simulink model "Controllers"  (R2024a)
settings: Solver=VariableStepAuto  StartTime=0.0  StopTime=10.0  RelTol=1e-3
undefined symbols (not defined in the file): Earth, gains, initcond, params, WGS84
libraries: ArdupilotFunctions x7, aerolibtransform2 x1, sharedtransform x1
settings Model: Creator=igmso  LastModifiedBy=igmso

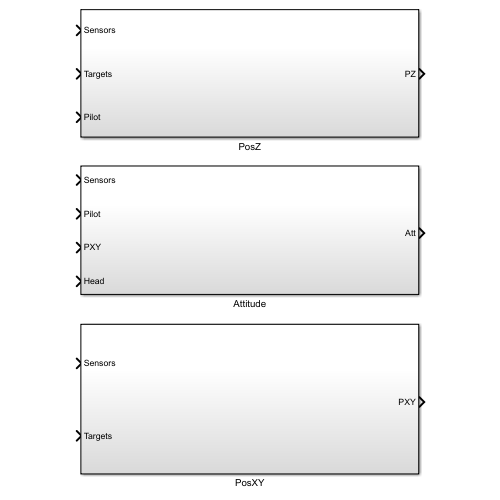
[thumbnail: Simulink's stored preview of the top-level diagram]
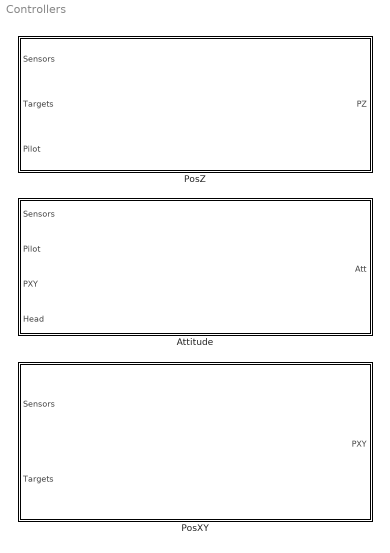
== system Controllers ==
  Attitude : Subsystem
  PosXY : Subsystem
  PosZ : Subsystem

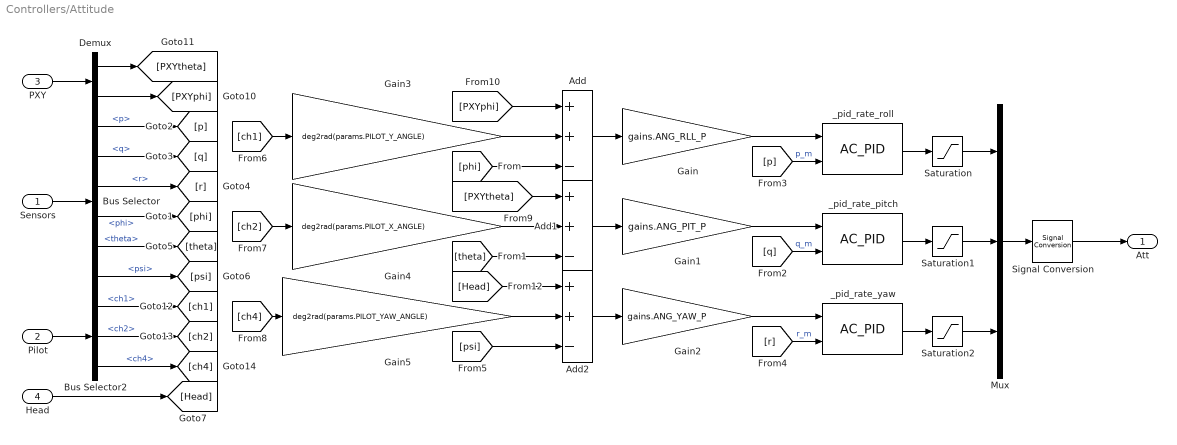
== system Controllers/Attitude ==
  Sensors : Inport  OutDataTypeStr=Bus: sensorsBus  PortDimensions=1
  Pilot : Inport  Port=2  OutDataTypeStr=Bus: pilotBus  PortDimensions=1
  PXY : Inport  Port=3  OutDataTypeStr=double  PortDimensions=2
  Head : Inport  Port=4  OutDataTypeStr=double  PortDimensions=1
  Add : Sum  Inputs=++-
  Add1 : Sum  Inputs=++-
  Add2 : Sum  Inputs=++-
  Bus Selector : BusSelector  OutputSignals=p,q,r,phi,theta,psi
  Bus Selector2 : BusSelector  OutputSignals=ch1,ch2,ch4
  Demux : Demux  Outputs=2
  Gain : Gain  Gain=gains.ANG_RLL_P
  Gain1 : Gain  Gain=gains.ANG_PIT_P
  Gain2 : Gain  Gain=gains.ANG_YAW_P
  Gain3 : Gain  Gain=deg2rad(params.PILOT_Y_ANGLE)
  Gain4 : Gain  Gain=deg2rad(params.PILOT_X_ANGLE)
  Gain5 : Gain  Gain=deg2rad(params.PILOT_YAW_ANGLE)
  Mux : Mux  Inputs=3
  Saturation : Saturate  UpperLimit=1  LowerLimit=-1
  Saturation1 : Saturate  UpperLimit=1  LowerLimit=-1
  Saturation2 : Saturate  UpperLimit=1  LowerLimit=-1
  Signal Conversion : SignalConversion  OverrideOpt=off
  _pid_rate_pitch : ArdupilotFunctions/AC_PID  P=gains.RAT_PIT_P  I=gains.RAT_PIT_I  D=gains.RAT_PIT_D  FF=gains.RAT_PIT_FF  D_FF=gains.RAT_PIT_D_FF  FLTD=gains.RAT_PIT_FLTD  FLTE=gains.RAT_PIT_FLTE  FLTT=gains.RAT_PIT_FLTT  IMAX=gains.RAT_PIT_IMAX  ControlFreq=rates.AttControl
  _pid_rate_roll : ArdupilotFunctions/AC_PID  P=gains.RAT_RLL_P  I=gains.RAT_RLL_I  D=gains.RAT_RLL_D  FF=gains.RAT_RLL_FF  D_FF=gains.RAT_RLL_D_FF  FLTD=gains.RAT_RLL_FLTD  FLTE=gains.RAT_RLL_FLTE  FLTT=gains.RAT_RLL_FLTT  IMAX=gains.RAT_RLL_IMAX  ControlFreq=rates.AttControl
  _pid_rate_yaw : ArdupilotFunctions/AC_PID  P=gains.RAT_YAW_P  I=gains.RAT_YAW_I  D=gains.RAT_YAW_D  FF=gains.RAT_YAW_FF  D_FF=gains.RAT_YAW_D_FF  FLTD=gains.RAT_YAW_FLTD  FLTE=gains.RAT_YAW_FLTE  FLTT=gains.RAT_YAW_FLTT  IMAX=gains.RAT_YAW_IMAX  ControlFreq=rates.AttControl
  Att : Outport  PortDimensions=3
  wires:
  Demux/1 -> [PXYtheta]
  _pid_rate_pitch/1 -> Saturation1/1
  Bus Selector2/3 -> [ch4]  "<ch4>"
  [ch2] -> Gain4/1
  Gain5/1 -> Add2/2
  Head/1 -> [Head]
  Bus Selector/2 -> [q]  "<q>"
  _pid_rate_roll/1 -> Saturation/1
  PXY/1 -> Demux/1
  [phi] -> Add/3
  Bus Selector/3 -> [r]  "<r>"
  [PXYtheta] -> Add1/1
  Bus Selector/5 -> [theta]  "<theta>"
  [Head] -> Add2/1
  Bus Selector/4 -> [phi]  "<phi>"
  Saturation2/1 -> Mux/3
  Gain4/1 -> Add1/2
  Mux/1 -> Signal Conversion/1
  [ch1] -> Gain3/1
  Gain2/1 -> _pid_rate_yaw/1
  Add2/1 -> Gain2/1
  [theta] -> Add1/3
  Signal Conversion/1 -> Att/1
  [q] -> _pid_rate_pitch/2  "q_m"
  Gain1/1 -> _pid_rate_pitch/1
  [p] -> _pid_rate_roll/2  "p_m"
  [r] -> _pid_rate_yaw/2  "r_m"
  [PXYphi] -> Add/1
  Add/1 -> Gain/1
  Sensors/1 -> Bus Selector/1
  [ch4] -> Gain5/1
  Gain3/1 -> Add/2
  Pilot/1 -> Bus Selector2/1
  Bus Selector/6 -> [psi]  "<psi>"
  Bus Selector/1 -> [p]  "<p>"
  Add1/1 -> Gain1/1
  Demux/2 -> [PXYphi]
  Saturation1/1 -> Mux/2
  _pid_rate_yaw/1 -> Saturation2/1
  Gain/1 -> _pid_rate_roll/1
  [psi] -> Add2/3
  Bus Selector2/2 -> [ch2]  "<ch2>"
  Bus Selector2/1 -> [ch1]  "<ch1>"
  Saturation/1 -> Mux/1

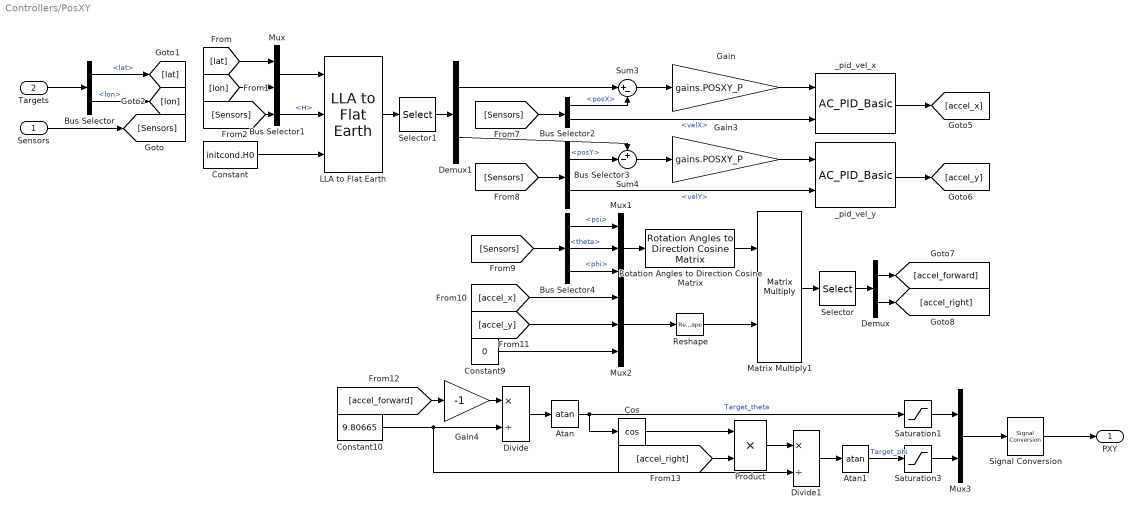
== system Controllers/PosXY ==
  Sensors : Inport  OutDataTypeStr=Bus: sensorsBus  PortDimensions=1
  Targets : Inport  Port=2  OutDataTypeStr=Bus: targetsBus  PortDimensions=1
  Atan : Trigonometry  Operator=atan
  Atan1 : Trigonometry  Operator=atan
  Bus Selector : BusSelector  OutputSignals=lat,lon
  Bus Selector1 : BusSelector  OutputSignals=H
  Bus Selector2 : BusSelector  OutputSignals=posX,velX
  Bus Selector3 : BusSelector  OutputSignals=posY,velY
  Bus Selector4 : BusSelector  OutputSignals=psi,theta,phi
  Constant : Constant  Value=initcond.H0  SampleTime=-1
  Constant10 : Constant  Value=9.80665  SampleTime=-1
  Constant9 : Constant  Value=0  SampleTime=-1
  Cos : Trigonometry  Operator=cos
  Demux : Demux  Outputs=2
  Demux1 : Demux  Outputs=2
  Divide : Product  Inputs=*/
  Divide1 : Product  Inputs=*/
  Gain : Gain  Gain=gains.POSXY_P
  Gain3 : Gain  Gain=gains.POSXY_P
  Gain4 : Gain  Gain=-1
  LLA to Flat Earth : aerolibtransform2/LLA to Flat Earth  units=Metric (MKS)  ptype=Earth (WGS84)  F=1/298.257223563  R=6378137  refPosPort=off  LL0=[0 10]  psi=0
  Matrix Multiply1 : Product  Multiplication=Matrix(*)
  Mux : Mux  Inputs=2
  Mux1 : Mux  Inputs=3
  Mux2 : Mux  Inputs=3
  Mux3 : Mux  Inputs=2
  Product : Product
  Reshape : Reshape  OutputDimensionality=Column vector (2-D)
  Rotation Angles to Direction Cosine Matrix : sharedtransform/Rotation Angles to Direction Cosine Matrix  rotationOrder=ZYX  aMode=aMode
  Saturation1 : Saturate  UpperLimit=deg2rad(gains.ANGLE_MAX)  LowerLimit=-deg2rad(gains.ANGLE_MAX)
  Saturation3 : Saturate
  Selector : Selector  InputPortWidth=3  IndexOptions=Index vector (dialog)  Indices=[1 2]  OutputSizes=1
  Selector1 : Selector  InputPortWidth=3  IndexOptions=Index vector (dialog)  Indices=[1 2]  OutputSizes=1
  Signal Conversion : SignalConversion  OverrideOpt=off
  Sum3 : Sum  Inputs=|+-
  Sum4 : Sum  Inputs=+-|
  _pid_vel_x : ArdupilotFunctions/AC_PID_Basic  P=gains.VELXY_P  I=gains.VELXY_I  D=gains.VELXY_D  FF=gains.VELXY_FF  FLTD=gains.VELXY_FLTD  FLTE=gains.VELXY_FLTE  IMAX=gains.VELXY_IMAX  ControlFreq=rates.PosControl
  _pid_vel_y : ArdupilotFunctions/AC_PID_Basic  P=gains.VELXY_P  I=gains.VELXY_I  D=gains.VELXY_D  FF=gains.VELXY_FF  FLTD=gains.VELXY_FLTD  FLTE=gains.VELXY_FLTE  IMAX=gains.VELXY_IMAX  ControlFreq=rates.PosControl
  PXY : Outport  PortDimensions=2
  wires:
  Reshape/1 -> Matrix Multiply1/2
  Saturation3/1 -> Mux3/2
  Divide/1 -> Atan/1
  Bus Selector/2 -> [lon]  "<lon>"
  Demux1/1 -> Sum3/1
  Sum3/1 -> Gain/1
  Bus Selector4/3 -> Mux1/3  "<phi>"
  Targets/1 -> Bus Selector/1
  Selector1/1 -> Demux1/1
  [Sensors] -> Bus Selector1/1
  _pid_vel_y/1 -> [accel_y]
  Product/1 -> Divide1/1
  Selector/1 -> Demux/1
  [Sensors] -> Bus Selector4/1
  Demux1/2 -> Sum4/1
  Gain/1 -> _pid_vel_x/1
  Mux1/1 -> Rotation Angles to Direction Cosine Matrix/1
  Sum4/1 -> Gain3/1
  Bus Selector3/2 -> _pid_vel_y/2  "<velY>"
  Bus Selector1/1 -> LLA to Flat Earth/2  "<H>"
  Divide1/1 -> Atan1/1
  Cos/1 -> Product/1
  [lat] -> Mux/1
  Constant10/1 -> Divide/2, Divide1/2
  Rotation Angles to Direction Cosine Matrix/1 -> Matrix Multiply1/1
  Saturation1/1 -> Mux3/1
  Sensors/1 -> [Sensors]
  Bus Selector2/1 -> Sum3/2  "<posX>"
  Atan1/1 -> Saturation3/1  "Target_phi"
  Bus Selector3/1 -> Sum4/2  "<posY>"
  _pid_vel_x/1 -> [accel_x]
  Demux/2 -> [accel_right]
  Bus Selector/1 -> [lat]  "<lat>"
  Gain3/1 -> _pid_vel_y/1
  Demux/1 -> [accel_forward]
  Constant/1 -> LLA to Flat Earth/3
  [Sensors] -> Bus Selector3/1
  [accel_right] -> Product/2
  Mux2/1 -> Reshape/1
  Atan/1 -> Cos/1, Saturation1/1  "Target_theta"
  Matrix Multiply1/1 -> Selector/1
  Mux3/1 -> Signal Conversion/1
  Mux/1 -> LLA to Flat Earth/1
  [accel_forward] -> Gain4/1
  Bus Selector4/2 -> Mux1/2  "<theta>"
  LLA to Flat Earth/1 -> Selector1/1
  [Sensors] -> Bus Selector2/1
  Bus Selector4/1 -> Mux1/1  "<psi>"
  Constant9/1 -> Mux2/3
  Bus Selector2/2 -> _pid_vel_x/2  "<velX>"
  Gain4/1 -> Divide/1
  Signal Conversion/1 -> PXY/1
  [accel_x] -> Mux2/1
  [lon] -> Mux/2
  [accel_y] -> Mux2/2

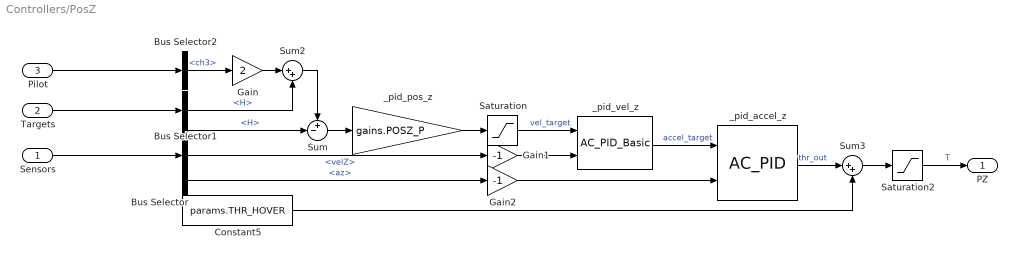
== system Controllers/PosZ ==
  Sensors : Inport  OutDataTypeStr=Bus: sensorsBus  PortDimensions=1
  Targets : Inport  Port=2  OutDataTypeStr=Bus: targetsBus  PortDimensions=1
  Pilot : Inport  Port=3  OutDataTypeStr=Bus: pilotBus  PortDimensions=1
  Bus Selector : BusSelector  OutputSignals=H,velZ,az
  Bus Selector1 : BusSelector  OutputSignals=H
  Bus Selector2 : BusSelector  OutputSignals=ch3
  Constant5 : Constant  Value=params.THR_HOVER  SampleTime=-1
  Gain : Gain  Gain=2
  Gain1 : Gain  Gain=-1
  Gain2 : Gain  Gain=-1
  Saturation : Saturate  UpperLimit=params.CLIMB_MAX  LowerLimit=-params.SINK_MAX
  Saturation2 : Saturate  UpperLimit=1  LowerLimit=0
  Sum : Sum  Inputs=+-|
  Sum2 : Sum  Inputs=|++
  Sum3 : Sum  Inputs=|++
  _pid_accel_z : ArdupilotFunctions/AC_PID  P=gains.ACCZ_P  I=gains.ACCZ_I  D=gains.ACCZ_D  FF=gains.ACCZ_FF*1e-3  D_FF=gains.ACCZ_D_FF*1e-3  FLTD=gains.ACCZ_FLTD  FLTE=gains.ACCZ_FLTE  FLTT=gains.ACCZ_FLTT  IMAX=gains.ACCZ_IMAX  ControlFreq=rates.PosControl
  _pid_pos_z : Gain  Gain=gains.POSZ_P
  _pid_vel_z : ArdupilotFunctions/AC_PID_Basic  P=gains.VELZ_P  I=gains.VELZ_I  D=gains.VELZ_D  FF=gains.VELZ_FF  FLTD=50  FLTE=50  IMAX=gains.VELZ_IMAX  ControlFreq=rates.PosControl
  PZ : Outport  OutDataTypeStr=double  PortDimensions=1
  wires:
  Bus Selector1/1 -> Sum2/2  "<H>"
  Bus Selector/3 -> Gain2/1  "<az>"
  Sum2/1 -> Sum/1
  Saturation/1 -> _pid_vel_z/1  "vel_target"
  Gain/1 -> Sum2/1
  Targets/1 -> Bus Selector1/1
  Constant5/1 -> Sum3/2
  Sum3/1 -> Saturation2/1
  _pid_pos_z/1 -> Saturation/1
  _pid_accel_z/1 -> Sum3/1  "thr_out"
  _pid_vel_z/1 -> _pid_accel_z/1  "accel_target"
  Sum/1 -> _pid_pos_z/1
  Gain2/1 -> _pid_accel_z/2
  Pilot/1 -> Bus Selector2/1
  Bus Selector2/1 -> Gain/1  "<ch3>"
  Bus Selector/2 -> Gain1/1  "<velZ>"
  Sensors/1 -> Bus Selector/1
  Gain1/1 -> _pid_vel_z/2
  Saturation2/1 -> PZ/1  "T"
  Bus Selector/1 -> Sum/2  "<H>"
